simulink model "Copy_of_Interleaved_parallel_buck"  (R2024b)
settings: Solver=VariableStepAuto  StartTime=0.0  StopTime=0.1  RelTol=1e-3
model workspace (MAT data in the model file):
  RC = 0
  RL = 0
  Ron = 1e-07
  f = 500000
libraries: spsCurrentMeasurementLib x9, spsMeanLib x9, spsVoltageMeasurementLib x6, spsSeriesRLCBranchLib x4, spsMosfetLib x4, spsRMSLib x4, slpidlib x2, eePowerMeasurement x2, spsSawtoothGeneratorLib x2, spsDCVoltageSourceLib x1, dspstat3 x1, sps_lib x1
settings Model: Creator=admin  LastModifiedBy=admin
settings SolverCC: AlgebraicLoopSolver=TrustRegion
settings DebuggingCC: UnconnectedInputMsg=warning  UnconnectedOutputMsg=warning  UnconnectedLineMsg=warning
settings ModelReferenceCC: EnableRefExpFcnMdlSchedulingChecks=on
settings RTWCC: GPUComputeCapability=3.5  DLArmComputeVersion=19.05

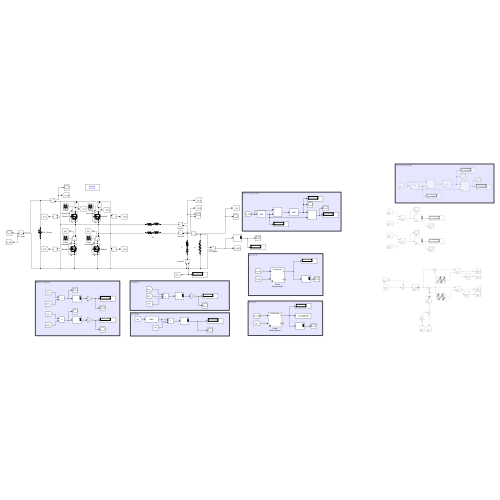
[thumbnail: Simulink's stored preview of the top-level diagram]
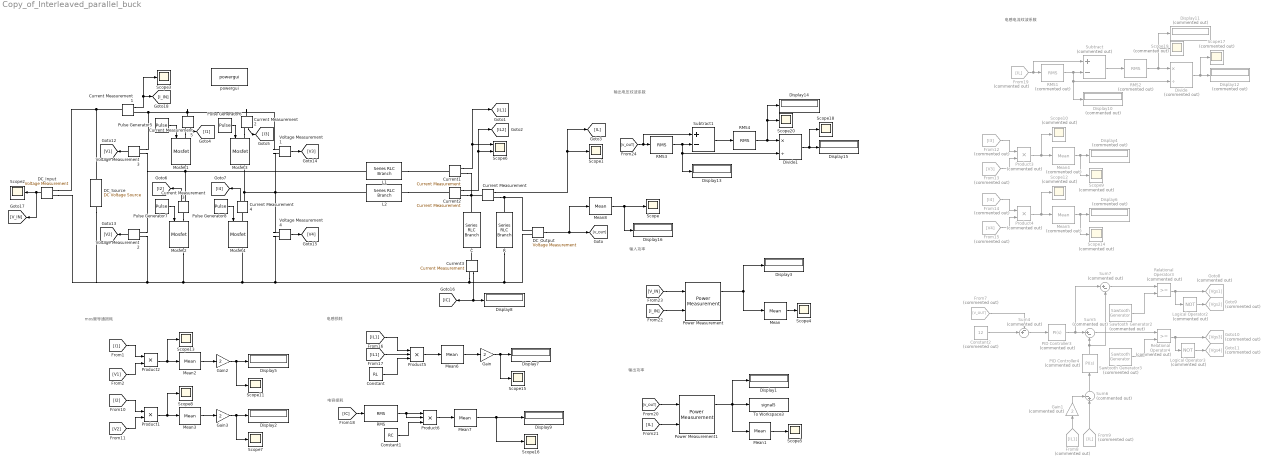
== system Copy_of_Interleaved_parallel_buck ==
  note: 电感电流纹波系数
  note: 输入功率
  note: 输出功率
  note: 电容损耗
  note: 电感损耗
  note: mos管导通损耗
  note: 输出电压纹波系数
  C : spsSeriesRLCBranchLib/Series RLC Branch  LConnTagsString=__new0  RConnTagsString=__new0  BranchType=RC  Resistance=RC  Inductance=1e-3  SetiL0=off  InitialCurrent=0  Capacitance=25/3/8/2/f/0.12  Setx0=off  InitialVoltage=0  Measurements=None
  Constant : Constant  Value=RL
  Constant1 : Constant  Value=RC
  Constant2 : Constant  Commented=on  Value=12
  Current Measurement{,1..5} (6 alike) : spsCurrentMeasurementLib/Current Measurement  PhasorSimulation=off  OutputType=Complex  PSBequivalent=0
  Current1 : spsCurrentMeasurementLib/Current Measurement  PhasorSimulation=off  OutputType=Complex  PSBequivalent=0
  Current2 : spsCurrentMeasurementLib/Current Measurement  PhasorSimulation=off  OutputType=Complex  PSBequivalent=0
  Current3 : spsCurrentMeasurementLib/Current Measurement  PhasorSimulation=off  OutputType=Complex  PSBequivalent=0
  DC_Input : spsVoltageMeasurementLib/Voltage Measurement  PhasorSimulation=off  OutputType=Complex  PSBequivalent=0
  DC_Output : spsVoltageMeasurementLib/Voltage Measurement  PhasorSimulation=off  OutputType=Complex  PSBequivalent=0
  DC_Source : spsDCVoltageSourceLib/DC Voltage Source  Amplitude=48  Measurements=None
  Display{1..3,5,7..9,13..16} (11 alike) : Display
  Display{4,6,10..12} (5 alike) : Display  Commented=on
  Divide : Product  Commented=on  Inputs=*/
  Divide1 : Product  Inputs=*/
  From12 : From  Commented=on  GotoTag=I3
  From13 : From  Commented=on  GotoTag=V3
  From14 : From  Commented=on  GotoTag=I4
  From15 : From  Commented=on  GotoTag=V4
  From19 : From  Commented=on  GotoTag=IL
  From7 : From  Commented=on  GotoTag=V_OUT
  From8 : From  Commented=on  GotoTag=IL1
  From9 : From  Commented=on  GotoTag=IL
  Gain : Gain  Gain=2
  Gain1 : Gain  Commented=on  Gain=2
  Gain2 : Gain  Gain=2
  Gain3 : Gain  Gain=2
  Goto10 : Goto  Commented=on  GotoTag=Vgs3
  Goto11 : Goto  Commented=on  GotoTag=Vgs4
  Goto8 : Goto  Commented=on  GotoTag=Vgs1
  Goto9 : Goto  Commented=on  GotoTag=Vgs2
  L1 : spsSeriesRLCBranchLib/Series RLC Branch  LConnTagsString=__new0  RConnTagsString=__new0  BranchType=RL  Resistance=RL  Inductance=36*12*3/48/f/25  SetiL0=off  InitialCurrent=0  Capacitance=1e-6  Setx0=off  InitialVoltage=0  Measurements=None
  L2 : spsSeriesRLCBranchLib/Series RLC Branch  LConnTagsString=__new0  RConnTagsString=__new0  BranchType=RL  Resistance=RL  Inductance=36*12*3/48/f/25  SetiL0=off  InitialCurrent=0  Capacitance=1e-6  Setx0=off  InitialVoltage=0  Measurements=None
  Logical Operator2 : Logic  Commented=on  Operator=NOT  AllPortsSameDT=off  OutDataTypeStr=boolean
  Logical Operator3 : Logic  Commented=on  Operator=NOT  AllPortsSameDT=off  OutDataTypeStr=boolean
  Mean{,1,7..8} (4 alike) : spsMeanLib/Mean  Freq=2*f  Vinit=0  Ts=0
  Mean2 : spsMeanLib/Mean  Freq=f  Vinit=0  Ts=0
  Mean3 : spsMeanLib/Mean  Freq=f  Vinit=0  Ts=0
  Mean4 : spsMeanLib/Mean  Commented=on  Freq=f  Vinit=0  Ts=0
  Mean5 : spsMeanLib/Mean  Commented=on  Freq=f  Vinit=0  Ts=0
  Mean6 : spsMeanLib/Mean  Freq=f  Vinit=0  Ts=0
  Mosfet{1..4} (4 alike) : spsMosfetLib/Mosfet  Ron=Ron  Lon=0  Rd=0.0001  Vfd=0  IC=0  Rs=1e5  Cs=inf  Measurements=on
  PID Controller3 : slpidlib/PID Controller  Commented=on  Controller=PI  Form=Parallel  TimeDomain=Continuous-time  UseExternalTs=off  SampleTime=-1  IntegratorMethod=Forward Euler  FilterMethod=Forward Euler  ControllerParametersSource=internal  P=0.1  I=5  UseKiTs=off  D=0  UseExternalDerivativeSource=off  N=100  UseFilter=on  TunerSelectOption=Transfer Function Based (PID Tuner App)  InitialConditionSource=internal  InitialConditionForIntegrator=0  InitialConditionForFilter=0  DifferentiatorICPrevScaledInput=0  ExternalReset=none  TrackingMode=off  Kt=1  LimitOutput=on  SatLimitsSource=internal  UpperSaturationLimit=4  LowerSaturationLimit=0.01  LinearizeAsGain=on  AntiWindupMode=none  Kb=1  LimitIntegrator=off  UpperIntegratorSaturationLimit=inf  LowerIntegratorSaturationLimit=-inf  POutMin=[]  POutMax=[]  IOutMin=[]  IOutMax=[]  DOutMin=[]  DOutMax=[]  NOutMin=[]  NOutMax=[]  SumOutMin=[]  SumOutMax=[]  SaturationOutMin=[]  SaturationOutMax=[]  PParamMin=[]  PParamMax=[]  IParamMin=[]  IParamMax=[]  DParamMin=[]  DParamMax=[]  NParamMin=[]  NParamMax=[]  KbParamMin=[]  KbParamMax=[]  KtParamMin=[]  KtParamMax=[]  KbOutMin=[]  KbOutMax=[]  KtOutMin=[]  KtOutMax=[]  IntegratorOutMin=[]  IntegratorOutMax=[]  FilterOutMin=[]  FilterOutMax=[]  SumI1OutMin=[]  SumI1OutMax=[]  SumI2OutMin=[]  SumI2OutMax=[]  SumI3OutMin=[]  SumI3OutMax=[]  SumI4OutMin=[]  SumI4OutMax=[]  SumDOutMin=[]  SumDOutMax=[]  DifferentiatorOutMin=[]  DifferentiatorOutMax=[]  FilterDiffOutCoefMin=[]  FilterDiffOutCoefMax=[]  ReciprocalOutMin=[]  ReciprocalOutMax=[]  SumDenOutMin=[]  SumDenOutMax=[]  SumNumOutMin=[]  SumNumOutMax=[]  DivideOutMin=[]  DivideOutMax=[]  UdiffTsProdOutMin=[]  UdiffTsProdOutMax=[]  NTsProdOutMin=[]  NTsProdOutMax=[]  UintegralTsProdOutMin=[]  UintegralTsProdOutMax=[]  UngainTsProdOutMin=[]  UngainTsProdOutMax=[]  ClampingZeroOutDataTypeStr=Inherit: Inherit via back propagation  ClampingZeroOutMin=[]  ClampingZeroOutMax=[]  FilterDenConstantOutDataTypeStr=Inherit: Inherit via back propagation  FilterDenConstantOutMin=[]  FilterDenConstantOutMax=[]  PCopyOutDataTypeStr=Inherit: Inherit via back propagation  PCopyOutMin=[]  PCopyOutMax=[]  NCopyOutDataTypeStr=Inherit: Inherit via back propagation  NCopyOutMin=[]  NCopyOutMax=[]  IntegratorContinuousStateAttributes=''  IntegratorStateMustResolveToSignalObject=off  IntegratorRTWStateStorageClass=Auto  FilterContinuousStateAttributes=''  FilterStateMustResolveToSignalObject=off  FilterRTWStateStorageClass=Auto  ParallelPVariant=InternalParameters  IdealPVariant=Disabled  IVariant=InternalParameters  DVariant=Disabled  IntegratorVariant=Continuous  SatVariant=Enabled  AWVariant=Passthrough  PCopyVariant=Disabled  TRVariant=Disabled  FdbkBlocksVariant=Forward  IdealPFdbkVariant=Disabled  SatFdbkVariant=Disabled  DerivativeFilterVariant=Disabled  NVariant=Disabled  NCopyVariant=Disabled_SignalSpec  FilterICVariant=Disabled  IntegratorICVariant=InternalICs  ExternalResetVariant=Disabled  TRSumVariant=Passthrough  SumFdbkVariant=Disabled  SumVariant=Sum_PI  TsampFilterVariant=InternalTs  TsampNgainVariant=Passthrough  TsampIntegralVariant=Passthrough  ExternalSaturationOutDataTypeStr=Inherit: Same as second input  DerivativeSourceVariant=ErrorSignal  PreIntVariant=InternalPreInt
  PID Controller4 : slpidlib/PID Controller  Commented=on  Controller=PI  Form=Parallel  TimeDomain=Continuous-time  UseExternalTs=off  SampleTime=-1  IntegratorMethod=Forward Euler  FilterMethod=Forward Euler  ControllerParametersSource=internal  P=0.1  I=30  UseKiTs=off  D=0  UseExternalDerivativeSource=off  N=100  UseFilter=on  TunerSelectOption=Transfer Function Based (PID Tuner App)  InitialConditionSource=internal  InitialConditionForIntegrator=0  InitialConditionForFilter=0  DifferentiatorICPrevScaledInput=0  ExternalReset=none  TrackingMode=off  Kt=1  LimitOutput=on  SatLimitsSource=internal  UpperSaturationLimit=0.95  LowerSaturationLimit=0.05  LinearizeAsGain=on  AntiWindupMode=none  Kb=1  LimitIntegrator=off  UpperIntegratorSaturationLimit=inf  LowerIntegratorSaturationLimit=-inf  POutMin=[]  POutMax=[]  IOutMin=[]  IOutMax=[]  DOutMin=[]  DOutMax=[]  NOutMin=[]  NOutMax=[]  SumOutMin=[]  SumOutMax=[]  SaturationOutMin=[]  SaturationOutMax=[]  PParamMin=[]  PParamMax=[]  IParamMin=[]  IParamMax=[]  DParamMin=[]  DParamMax=[]  NParamMin=[]  NParamMax=[]  KbParamMin=[]  KbParamMax=[]  KtParamMin=[]  KtParamMax=[]  KbOutMin=[]  KbOutMax=[]  KtOutMin=[]  KtOutMax=[]  IntegratorOutMin=[]  IntegratorOutMax=[]  FilterOutMin=[]  FilterOutMax=[]  SumI1OutMin=[]  SumI1OutMax=[]  SumI2OutMin=[]  SumI2OutMax=[]  SumI3OutMin=[]  SumI3OutMax=[]  SumI4OutMin=[]  SumI4OutMax=[]  SumDOutMin=[]  SumDOutMax=[]  DifferentiatorOutMin=[]  DifferentiatorOutMax=[]  FilterDiffOutCoefMin=[]  FilterDiffOutCoefMax=[]  ReciprocalOutMin=[]  ReciprocalOutMax=[]  SumDenOutMin=[]  SumDenOutMax=[]  SumNumOutMin=[]  SumNumOutMax=[]  DivideOutMin=[]  DivideOutMax=[]  UdiffTsProdOutMin=[]  UdiffTsProdOutMax=[]  NTsProdOutMin=[]  NTsProdOutMax=[]  UintegralTsProdOutMin=[]  UintegralTsProdOutMax=[]  UngainTsProdOutMin=[]  UngainTsProdOutMax=[]  ClampingZeroOutDataTypeStr=Inherit: Inherit via back propagation  ClampingZeroOutMin=[]  ClampingZeroOutMax=[]  FilterDenConstantOutDataTypeStr=Inherit: Inherit via back propagation  FilterDenConstantOutMin=[]  FilterDenConstantOutMax=[]  PCopyOutDataTypeStr=Inherit: Inherit via back propagation  PCopyOutMin=[]  PCopyOutMax=[]  NCopyOutDataTypeStr=Inherit: Inherit via back propagation  NCopyOutMin=[]  NCopyOutMax=[]  IntegratorContinuousStateAttributes=''  IntegratorStateMustResolveToSignalObject=off  IntegratorRTWStateStorageClass=Auto  FilterContinuousStateAttributes=''  FilterStateMustResolveToSignalObject=off  FilterRTWStateStorageClass=Auto  ParallelPVariant=InternalParameters  IdealPVariant=Disabled  IVariant=InternalParameters  DVariant=Disabled  IntegratorVariant=Continuous  SatVariant=Enabled  AWVariant=Passthrough  PCopyVariant=Disabled  TRVariant=Disabled  FdbkBlocksVariant=Forward  IdealPFdbkVariant=Disabled  SatFdbkVariant=Disabled  DerivativeFilterVariant=Disabled  NVariant=Disabled  NCopyVariant=Disabled_SignalSpec  FilterICVariant=Disabled  IntegratorICVariant=InternalICs  ExternalResetVariant=Disabled  TRSumVariant=Passthrough  SumFdbkVariant=Disabled  SumVariant=Sum_PI  TsampFilterVariant=InternalTs  TsampNgainVariant=Passthrough  TsampIntegralVariant=Passthrough  ExternalSaturationOutDataTypeStr=Inherit: Same as second input  DerivativeSourceVariant=ErrorSignal  PreIntVariant=InternalPreInt
  Power Measurement : eePowerMeasurement/Power Measurement  LabelModeActiveChoice=Continuous  F=60  K=[0]  Ts=0
  Power Measurement1 : eePowerMeasurement/Power Measurement  LabelModeActiveChoice=Continuous  F=60  K=[0]  Ts=0
  Product1 : Product
  Product2 : Product
  Product3 : Product  Commented=on
  Product4 : Product  Commented=on
  Product5 : Product  Inputs=3
  Product6 : Product  Inputs=3
  Pulse Generator5 : DiscretePulseGenerator  PulseType=Time based  Period=1/f  PulseWidth=25
  Pulse Generator6 : DiscretePulseGenerator  PulseType=Time based  Period=1/f  PulseWidth=25  PhaseDelay=2/4/f
  Pulse Generator7 : DiscretePulseGenerator  PulseType=Time based  Period=1/f  PulseWidth=25  PhaseDelay=1/4/f
  Pulse Generator8 : DiscretePulseGenerator  PulseType=Time based  Period=1/f  PulseWidth=25  PhaseDelay=3/4/f
  R : spsSeriesRLCBranchLib/Series RLC Branch  LConnTagsString=__new0  RConnTagsString=__new0  BranchType=R  Resistance=0.072  Inductance=1e-3  SetiL0=off  InitialCurrent=0  Capacitance=1e-6  Setx0=off  InitialVoltage=0  Measurements=None
  RMS : dspstat3/RMS  run=off  directionMode=Each column  dimension=1  InputProcessing=Columns as channels (frame based)  reset_popup=None
  RMS1 : spsRMSLib/RMS  Commented=on  TrueRMS=on  Freq=60  RMSInit=0  Ts=0
  RMS2 : spsRMSLib/RMS  Commented=on  TrueRMS=on  Freq=60  RMSInit=0  Ts=0
  RMS3 : spsRMSLib/RMS  TrueRMS=on  Freq=60  RMSInit=0  Ts=0
  RMS4 : spsRMSLib/RMS  TrueRMS=on  Freq=60  RMSInit=0  Ts=0
  Relational Operator3 : RelationalOperator  Commented=on  OutDataTypeStr=boolean  RndMeth=Simplest  InputSameDT=off
  Relational Operator4 : RelationalOperator  Commented=on  OutDataTypeStr=boolean  RndMeth=Simplest  InputSameDT=off
  Sawtooth Generator2 : spsSawtoothGeneratorLib/Sawtooth Generator  Commented=on  Freq=1000e3  Phase=0  Ts=0
  Sawtooth Generator3 : spsSawtoothGeneratorLib/Sawtooth Generator  Commented=on  Freq=1000e3  Phase=180  Ts=0
  Scope{,1..5,7..8,11,13,15..16,18,20} (14 alike) : Scope
  Scope{9..10,12,14,17,19} (6 alike) : Scope  Commented=on
  Scope6 : Scope  NumInputPorts=2
  Subtract : Sum  Commented=on  Inputs=+-
  Subtract1 : Sum  Inputs=+-
  Sum4 : Sum  Commented=on  Inputs=-+|
  Sum5 : Sum  Commented=on  Inputs=|+-
  Sum6 : Sum  Commented=on  Inputs=-+|
  Sum7 : Sum  Commented=on  Inputs=|+-
  To Workspace3 : ToWorkspace  VariableName=signal5  SampleTime=0.1
  Voltage Measurement{1..4} (4 alike) : spsVoltageMeasurementLib/Voltage Measurement  PhasorSimulation=off  OutputType=Complex  PSBequivalent=0
  powergui : sps_lib/powergui  Priority=1  SimulationMode=Discrete  SampleTime=5e-8  frequency=60  Iterations=50  frequencyindice=0  Pbase=100e6  ErrMax=1e-4  UnitsV=kV  UnitsW=MW  buscounter=0  FunctionMessages=off  echomessages=off  EnableUseOfTLC=off  CurrentSourceSwitches=off  DisableSnubberDevices=off  DisableRonSwitches=off  DisableVfSwitches=off  DisplayEquations=off  AutomaticDiscreteSolvers=off  SolverType=Tustin/Backward Euler (TBE)  Interpol=off  ExternalGateDelay=off  methode=off  Ts=100  x0status=blocks  SPID=on  SwTol=0  HookPort=off  NonlinearTolerance=1e-4  nMaxIteration=100  ContinueOnMaxIteration=off  RestoreLinks=warning  ResistiveCurrentMeasurement=off  Frange=[0:2:500]  Ylog=off  Xlog=on  ShowGrid=off  save=off  variable=ZData  structure=0  ZoomFFT=off  StartTime=0.0  cycles=1  DisplayStyle=1  fundamental=60  FreqAxis=off  MaxFrequency=1000  frequencyindicesteady=1  RmsSteady=1  display=off
  wires:
  DC_Output/1 -> Mean8/1, [V_OUT]
  DC_Input/1 -> [V_IN], Scope2/1
  Current Measurement/1 -> [IL], Scope1/1
  Current1/1 -> [IL1], Scope6/1
  Current2/1 -> [IL2], Scope6/2
  Constant2/1 -> Sum4/2
  From7/1 -> Sum4/1
  Sum4/1 -> PID Controller3/1
  PID Controller3/1 -> Sum7/1, Sum5/1
  Gain1/1 -> Sum6/1
  From8/1 -> Gain1/1
  From9/1 -> Sum6/2
  Sum6/1 -> PID Controller4/1
  PID Controller4/1 -> Sum7/2, Sum5/2
  Sum7/1 -> Relational Operator3/1
  Sawtooth Generator2/1 -> Relational Operator3/2
  Sum5/1 -> Relational Operator4/1
  Sawtooth Generator3/1 -> Relational Operator4/2
  Logical Operator2/1 -> Goto9/1
  Relational Operator3/1 -> Logical Operator2/1, Goto8/1
  Logical Operator3/1 -> Goto11/1
  Relational Operator4/1 -> Logical Operator3/1, Goto10/1
  Pulse Generator5/1 -> Mosfet1/1
  Pulse Generator6/1 -> Mosfet3/1
  Pulse Generator8/1 -> Mosfet4/1
  Pulse Generator7/1 -> Mosfet2/1
  Mean/1 -> Scope4/1
  Power Measurement/1 -> Display3/1, Mean/1
  Current Measurement5/1 -> [I1]
  Current Measurement2/1 -> [I3]
  Current Measurement3/1 -> [I2]
  Current Measurement4/1 -> [I4]
  Voltage Measurement3/1 -> [V1]
  Voltage Measurement1/1 -> [V3]
  Voltage Measurement4/1 -> [V4]
  Voltage Measurement2/1 -> [V2]
  Power Measurement1/1 -> Mean1/1, Display1/1, To Workspace3/1
  Mean1/1 -> Scope5/1
  [I1] -> Product2/1
  [V1] -> Product2/2
  Product2/1 -> Mean2/1, Scope13/1
  Product1/1 -> Scope8/1, Mean3/1
  [V2] -> Product1/2
  [I2] -> Product1/1
  From12/1 -> Product3/1
  From13/1 -> Product3/2
  Product3/1 -> Mean4/1, Scope10/1
  Mean4/1 -> Scope9/1, Display4/1
  Mean5/1 -> Display6/1, Scope14/1
  Product4/1 -> Scope12/1, Mean5/1
  From15/1 -> Product4/2
  From14/1 -> Product4/1
  [IL1] -> Product5/1
  [IL1] -> Product5/2
  Constant/1 -> Product5/3
  Product5/1 -> Mean6/1
  Mean6/1 -> Gain/1
  Gain/1 -> Scope15/1, Display7/1
  Current3/1 -> [IC], Display8/1
  [IC] -> RMS/1
  Constant1/1 -> Product6/3
  Product6/1 -> Mean7/1
  Mean7/1 -> Scope16/1, Display9/1
  Mean2/1 -> Gain2/1
  Gain2/1 -> Scope11/1, Display5/1
  Mean3/1 -> Gain3/1
  Gain3/1 -> Scope7/1, Display2/1
  [V_OUT] -> Power Measurement1/1
  [IL] -> Power Measurement1/2
  Current Measurement1/1 -> Scope3/1, [I_IN]
  [I_IN] -> Power Measurement/2
  [V_IN] -> Power Measurement/1
  RMS/1 -> Product6/2, Product6/1
  From19/1 -> Subtract/1, RMS1/1
  RMS1/1 -> Subtract/2, Divide/2, Display10/1
  Subtract/1 -> RMS2/1
  RMS2/1 -> Divide/1, Scope19/1, Display11/1
  Divide/1 -> Scope17/1, Display12/1
  Divide1/1 -> Display15/1, Scope18/1
  RMS4/1 -> Scope20/1, Display14/1, Divide1/1
  Subtract1/1 -> RMS4/1
  RMS3/1 -> Display13/1, Divide1/2, Subtract1/2
  [V_OUT] -> RMS3/1, Subtract1/1
  Mean8/1 -> Display16/1, Scope/1
  connections:
  Mosfet1/RConn1 -- Voltage Measurement2/LConn2 -- Voltage Measurement3/LConn2 -- Current Measurement3/RConn1 -- L1/LConn1
  Current Measurement5/LConn1 -- Current Measurement2/LConn1 -- Voltage Measurement1/LConn1 -- Voltage Measurement3/LConn1 -- Current Measurement1/RConn1
  R/RConn1 -- DC_Output/LConn2 -- Current3/RConn1 -- Voltage Measurement4/LConn1 -- Mosfet2/RConn1 -- Voltage Measurement2/LConn1 -- DC_Source/LConn1 -- DC_Input/LConn2 -- Mosfet4/RConn1
  DC_Source/RConn1 -- DC_Input/LConn1 -- Current Measurement1/LConn1
  L2/LConn1 -- Voltage Measurement4/LConn2 -- Mosfet3/RConn1 -- Current Measurement4/RConn1 -- Voltage Measurement1/LConn2
  C/LConn1 -- Current1/RConn1 -- Current Measurement/LConn1 -- Current2/RConn1
  Current Measurement/RConn1 -- DC_Output/LConn1 -- R/LConn1
  L2/RConn1 -- Current2/LConn1
  L1/RConn1 -- Current1/LConn1
  Current Measurement5/RConn1 -- Mosfet1/LConn1
  Current Measurement2/RConn1 -- Mosfet3/LConn1
  Current Measurement3/LConn1 -- Mosfet2/LConn1
  Mosfet4/LConn1 -- Current Measurement4/LConn1
  Current3/LConn1 -- C/RConn1
